simulink model "SCS_MotorGearLeadScrew"  (R2026a)
settings: Solver=ode4  StopTime=80  FixedStep=0.0005
values from neighbouring files (symbols this model uses):
  B = 0.001    [build_motor_alone_model.m]    (also in build_motor_gearleadscrew_model.m; run_motor_alone_tests.m; run_motor_gearleadscrew_tests.m)
  gearEfficiency = 0.85    [build_motor_gearleadscrew_model.m]    (also in run_motor_gearleadscrew_tests.m)
  gearRatio = 5    [build_motor_gearleadscrew_model.m]    (also in run_motor_gearleadscrew_tests.m)
  J = 0.0005    [build_motor_alone_model.m]    (also in build_motor_gearleadscrew_model.m; run_motor_alone_tests.m; run_motor_gearleadscrew_tests.m)
  Ke = 0.05    [build_motor_alone_model.m]    (also in build_motor_gearleadscrew_model.m; run_motor_alone_tests.m; run_motor_gearleadscrew_tests.m)
  Kt = 0.05    [build_motor_alone_model.m]    (also in build_motor_gearleadscrew_model.m; run_motor_alone_tests.m; run_motor_gearleadscrew_tests.m)
  L = 0.005    [build_motor_alone_model.m]    (also in build_motor_gearleadscrew_model.m; run_motor_alone_tests.m; run_motor_gearleadscrew_tests.m)
  R = 2    [build_motor_alone_model.m]    (also in build_motor_gearleadscrew_model.m; run_motor_alone_tests.m; run_motor_gearleadscrew_tests.m)
  screwPitch = 4    [build_motor_gearleadscrew_model.m]    (also in run_motor_gearleadscrew_tests.m)
settings Model: Creator=singh  LastModifiedBy=singh

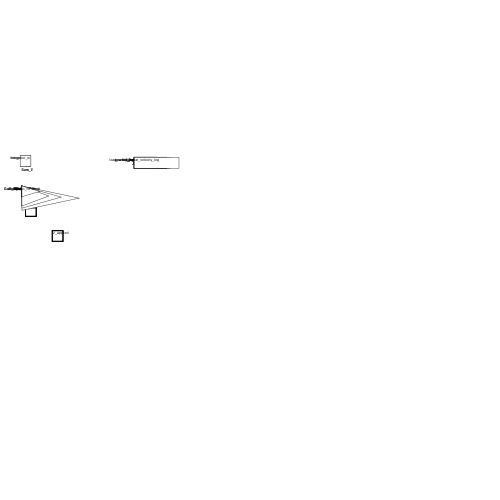
[thumbnail: Simulink's stored preview of the top-level diagram]
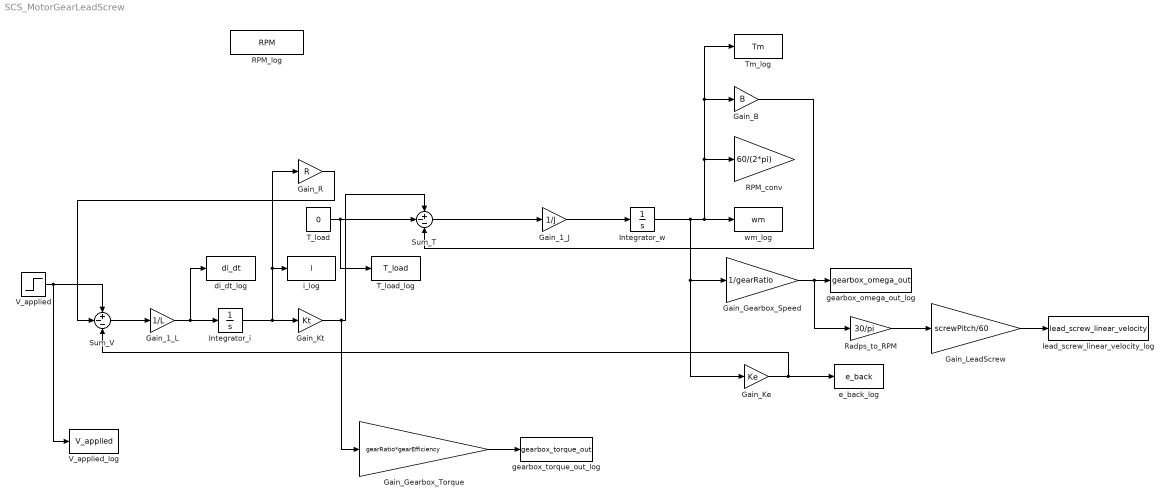
== system SCS_MotorGearLeadScrew ==
  Gain_1_J : Gain  Gain=1/J
  Gain_1_L : Gain  Gain=1/L
  Gain_B : Gain  Gain=B
  Gain_Gearbox_Speed : Gain  Gain=1/gearRatio
  Gain_Gearbox_Torque : Gain  Gain=gearRatio*gearEfficiency
  Gain_Ke : Gain  Gain=Ke
  Gain_Kt : Gain  Gain=Kt
  Gain_LeadScrew : Gain  Gain=screwPitch/60
  Gain_R : Gain  Gain=R
  Integrator_i : Integrator
  Integrator_w : Integrator
  RPM_conv : Gain  Gain=60/(2*pi)
  RPM_log : ToWorkspace  VariableName=RPM  SaveFormat=Structure With Time  SampleTime=-1
  Radps_to_RPM : Gain  Gain=30/pi
  Sum_T : Sum  Inputs=+--
  Sum_V : Sum  Inputs=+--
  T_load : Constant  Value=0
  T_load_log : ToWorkspace  VariableName=T_load  SaveFormat=Structure With Time  SampleTime=-1
  Tm_log : ToWorkspace  VariableName=Tm  SaveFormat=Structure With Time  SampleTime=-1
  V_applied : Step  FinalValue=9.42  SampleTime=0
  V_applied_log : ToWorkspace  VariableName=V_applied  SaveFormat=Structure With Time  SampleTime=-1
  di_dt_log : ToWorkspace  VariableName=di_dt  SaveFormat=Structure With Time  SampleTime=-1
  e_back_log : ToWorkspace  VariableName=e_back  SaveFormat=Structure With Time  SampleTime=-1
  gearbox_omega_out_log : ToWorkspace  VariableName=gearbox_omega_out  SaveFormat=Structure With Time  SampleTime=-1
  gearbox_torque_out_log : ToWorkspace  VariableName=gearbox_torque_out  SaveFormat=Structure With Time  SampleTime=-1
  i_log : ToWorkspace  VariableName=i  SaveFormat=Structure With Time  SampleTime=-1
  lead_screw_linear_velocity_log : ToWorkspace  VariableName=lead_screw_linear_velocity  SaveFormat=Structure With Time  SampleTime=-1
  wm_log : ToWorkspace  VariableName=wm  SaveFormat=Structure With Time  SampleTime=-1
  wires:
  Gain_LeadScrew/1 -> lead_screw_linear_velocity_log/1
  Radps_to_RPM/1 -> Gain_LeadScrew/1
  Gain_Ke/1 -> e_back_log/1, Sum_V/3
  V_applied/1 -> V_applied_log/1, Sum_V/1
  Gain_R/1 -> Sum_V/2
  T_load/1 -> T_load_log/1, Sum_T/2
  Gain_Kt/1 -> Gain_Gearbox_Torque/1, Sum_T/1
  Sum_V/1 -> Gain_1_L/1
  Sum_T/1 -> Gain_1_J/1
  Gain_1_J/1 -> Integrator_w/1
  Gain_Gearbox_Speed/1 -> Radps_to_RPM/1, gearbox_omega_out_log/1
  Integrator_i/1 -> i_log/1, Gain_R/1, Gain_Kt/1
  Gain_Gearbox_Torque/1 -> gearbox_torque_out_log/1
  Gain_1_L/1 -> di_dt_log/1, Integrator_i/1
  Gain_B/1 -> Sum_T/3
  Integrator_w/1 -> Gain_Gearbox_Speed/1, Gain_Ke/1, Tm_log/1, Gain_B/1, RPM_conv/1, wm_log/1
